simulink model "figure_4_temperature_control_block"  (R2021a)
settings: Solver=VariableStepAuto  StartTime=0.0  StopTime=10.0  RelTol=1e-3
model workspace (MAT data in the model file):
  K4 = Simulink.Parameter
  K4.DataType = 'auto'
  K4.Dimensions = [0 0]
  K5 = Simulink.Parameter
  K5.DataType = 'auto'
  K5.Dimensions = [0 0]
  T3 = Simulink.Parameter
  T3.DataType = 'auto'
  T3.Dimensions = [0 0]
  T4 = Simulink.Parameter
  T4.DataType = 'auto'
  T4.Dimensions = [0 0]
  T5 = Simulink.Parameter
  T5.DataType = 'auto'
  T5.Dimensions = [0 0]
  Teo = Simulink.Parameter
  Teo.DataType = 'auto'
  Teo.Dimensions = [0 0]
  Tt = Simulink.Parameter
  Tt.DataType = 'auto'
  Tt.Dimensions = [0 0]
settings Model: Creator=Souvik Datta  LastModifiedBy=user

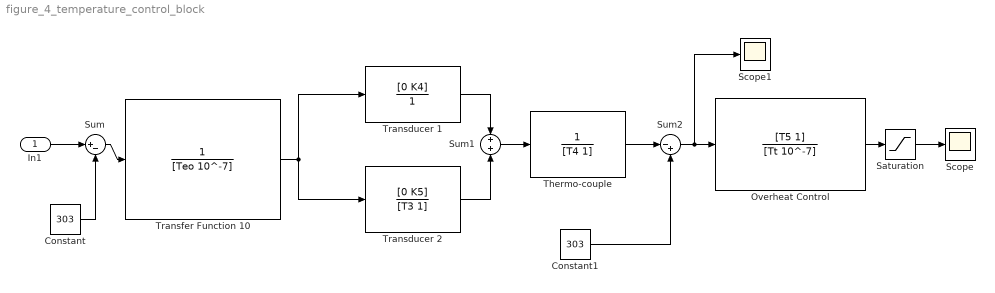
== system figure_4_temperature_control_block ==
  In1 : Inport
  Constant : Constant  Value=303
  Constant1 : Constant  Value=303
  Overheat Control : TransferFcn  Numerator=[T5 1]  Denominator=[Tt 10^-7]
  Saturation : Saturate  UpperLimit=350
  Scope : Scope
  Scope1 : Scope
  Sum : Sum  Inputs=|+-
  Sum1 : Sum  Inputs=+|+
  Sum2 : Sum  Inputs=|-+
  Thermo-couple : TransferFcn  Denominator=[T4 1]
  Transducer 1 : TransferFcn  Numerator=[0 K4]  Denominator=[0 1]
  Transducer 2 : TransferFcn  Numerator=[0 K5]  Denominator=[T3 1]
  Transfer Function 10 : TransferFcn  Denominator=[Teo 10^-7]
  wires:
  Constant/1 -> Sum/2
  In1/1 -> Sum/1
  Sum/1 -> Transfer Function 10/1
  Transfer Function 10/1 -> Transducer 1/1, Transducer 2/1
  Transducer 2/1 -> Sum1/2
  Transducer 1/1 -> Sum1/1
  Sum1/1 -> Thermo-couple/1
  Constant1/1 -> Sum2/2
  Thermo-couple/1 -> Sum2/1
  Sum2/1 -> Scope1/1, Overheat Control/1
  Overheat Control/1 -> Saturation/1
  Saturation/1 -> Scope/1
